simulink model "PaulPF"  (R2017a)
settings: Solver=FixedStepAuto  StartTime=0.0  StopTime=0.1  FixedStep=1/10e6  RelTol=1e-3
libraries: cstblocks x1
settings Model: Creator=bhannigan  LastModifiedBy=bhannigan

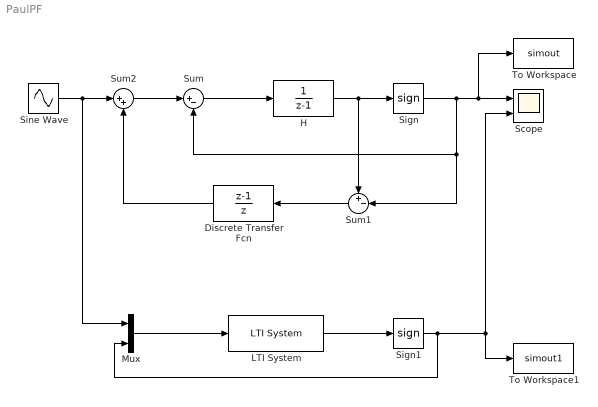
== system PaulPF ==
  Discrete Transfer Fcn : DiscreteTransferFcn  Numerator=[1 -1]  Denominator=[1 0]
  H : DiscreteTransferFcn  Numerator=1  Denominator=[1 -1]
  LTI System : cstblocks/LTI System  sys=sys  IC=[]
  Mux : Mux  Inputs=2
  Scope : Scope  NumInputPorts=2
  Sign : Signum
  Sign1 : Signum
  Sine Wave : Sin  Frequency=2*pi*1000  SampleTime=0
  Sum : Sum  Inputs=|+-
  Sum1 : Sum  Inputs=+-|
  Sum2 : Sum  Inputs=|++
  To Workspace : ToWorkspace  VariableName=simout  SaveFormat=Timeseries  SampleTime=-1
  To Workspace1 : ToWorkspace  VariableName=simout1  SaveFormat=Timeseries  SampleTime=-1
  wires:
  Sum/1 -> H/1
  H/1 -> Sum1/1, Sign/1
  Sign/1 -> To Workspace/1, Scope/1, Sum/2, Sum1/2
  Sum1/1 -> Discrete Transfer Fcn/1
  Sine Wave/1 -> Mux/1, Sum2/1
  Sum2/1 -> Sum/1
  Discrete Transfer Fcn/1 -> Sum2/2
  Mux/1 -> LTI System/1
  LTI System/1 -> Sign1/1
  Sign1/1 -> Mux/2, To Workspace1/1, Scope/2
